simulink model "newrules"  (R2016a)
settings: Solver=VariableStepAuto  StartTime=0.0  StopTime=10.0  RelTol=1e-3
libraries: fuzblock x5, simulink x1
settings Model: Creator=SPDKH  LastModifiedBy=SPDKH

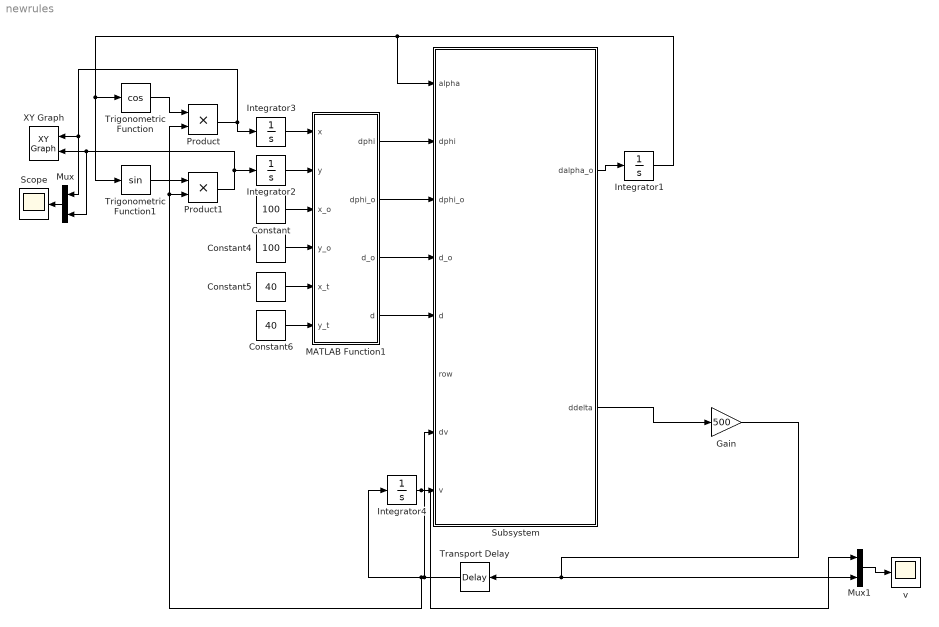
== system newrules ==
  Constant : Constant  Value=100
  Constant4 : Constant  Value=100
  Constant5 : Constant  Value=40
  Constant6 : Constant  Value=40
  Gain : Gain  Gain=500
  Integrator1 : Integrator
  Integrator2 : Integrator
  Integrator3 : Integrator  InitialCondition=30
  Integrator4 : Integrator
  MATLAB Function1 : MATLAB Function  TreatAsAtomicUnit=on
  Mux : Mux  Inputs=2
  Mux1 : Mux  Inputs=2
  Product : Product
  Product1 : Product
  Scope : Scope
  Subsystem : Subsystem
  Transport Delay : TransportDelay
  Trigonometric Function : Trigonometry  Operator=cos
  Trigonometric Function1 : Trigonometry
  XY Graph : simulink/Sinks/XY Graph  xmin=-10  xmax=100  ymin=-10  ymax=100  st=-1
  v : Scope
  wires:
  Subsystem/2(ddelta) -> Gain/1
  Constant/1 -> MATLAB Function1/3(x_o)
  Constant4/1 -> MATLAB Function1/4(y_o)
  Constant5/1 -> MATLAB Function1/5(x_t)
  Constant6/1 -> MATLAB Function1/6(y_t)
  MATLAB Function1/1(dphi) -> Subsystem/2("dphi ")
  MATLAB Function1/2(dphi_o) -> Subsystem/3("dphi_o ")
  MATLAB Function1/3(d_o) -> Subsystem/4(d_o)
  MATLAB Function1/4(d) -> Subsystem/5(d)
  Subsystem/1("dalpha_o ") -> Integrator1/1
  Integrator2/1 -> MATLAB Function1/2(y)
  Integrator3/1 -> MATLAB Function1/1(x)
  Trigonometric Function/1 -> Product/1
  Trigonometric Function1/1 -> Product1/1
  Integrator1/1 -> Subsystem/1(alpha), Trigonometric Function1/1, Trigonometric Function/1
  Product/1 -> Mux/1, XY Graph/1, Integrator3/1
  Product1/1 -> Mux/2, XY Graph/2, Integrator2/1
  Gain/1 -> Mux1/2, Transport Delay/1
  Transport Delay/1 -> Integrator4/1, Product1/2, Product/2, Subsystem/7(dv)
  Mux1/1 -> v/1
  Integrator4/1 -> Mux1/1, Subsystem/8(v)
  Mux/1 -> Scope/1

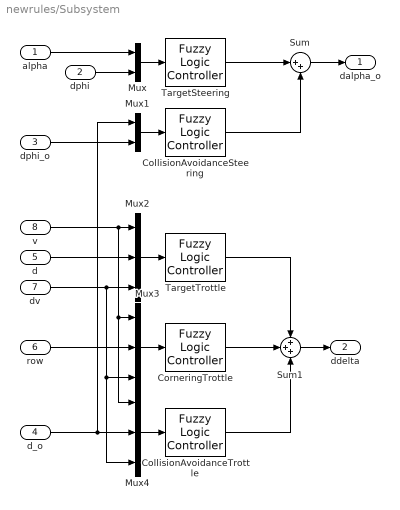
== system newrules/Subsystem ==
  alpha : Inport
  "dphi " : Inport  Port=2
  "dphi_o " : Inport  Port=3
  d_o : Inport  Port=4
  d : Inport  Port=5
  row : Inport  Port=6
  dv : Inport  Port=7
  v : Inport  Port=8
  "CollisionAvoidanceSteering " : fuzblock/Fuzzy Logic  Controller  fis=['CollisionAvoidanceSteering.fis']
  "CollisionAvoidanceTrottle " : fuzblock/Fuzzy Logic  Controller  fis=['CollisionAvoidanceThrottle.fis']
  "CorneringTrottle " : fuzblock/Fuzzy Logic  Controller  fis=['CorneringTrottle.fis']
  Mux : Mux  Inputs=2
  Mux1 : Mux  Inputs=2
  Mux2 : Mux  Inputs=3
  Mux3 : Mux  Inputs=3
  Mux4 : Mux  Inputs=3
  Sum : Sum  Inputs=|++
  Sum1 : Sum  Inputs=+++
  TargetSteering : fuzblock/Fuzzy Logic  Controller  fis=['TargetSteering2.fis']
  TargetTrottle : fuzblock/Fuzzy Logic  Controller  fis=['TargetTrottle.fis']
  "dalpha_o " : Outport
  ddelta : Outport  Port=2
  wires:
  TargetTrottle/1 -> Sum1/1
  "CorneringTrottle "/1 -> Sum1/2
  "CollisionAvoidanceTrottle "/1 -> Sum1/3
  TargetSteering/1 -> Sum/1
  "CollisionAvoidanceSteering "/1 -> Sum/2
  Mux/1 -> TargetSteering/1
  Mux1/1 -> "CollisionAvoidanceSteering "/1
  Mux2/1 -> TargetTrottle/1
  Mux3/1 -> "CorneringTrottle "/1
  Mux4/1 -> "CollisionAvoidanceTrottle "/1
  v/1 -> Mux4/1, Mux3/1, Mux2/1
  d/1 -> Mux2/2
  dv/1 -> Mux4/3, Mux3/3, Mux2/3
  row/1 -> Mux3/2
  d_o/1 -> Mux1/1, Mux4/2
  alpha/1 -> Mux/1
  "dphi "/1 -> Mux/2
  "dphi_o "/1 -> Mux1/2
  Sum/1 -> "dalpha_o "/1
  Sum1/1 -> ddelta/1

== matlab function newrules/MATLAB Function1 ==
  data: dphi output; dphi_o output; d_o output; x input; d output; y input; x_o input; y_o input; x_t input; y_t input
function [dphi,dphi_o,d_o,d] = fcn(x,y,x_o,y_o,x_t,y_t)

 if ((x_t-x) < 0)
     dphi = atan ((y_t-y)/(x_t-x))+pi;
 else 
    dphi = atan ((y_t-y)/(x_t-x));
 end
 
 if ((x_o-x) < 0)
     dphi_o = atan ((y_o-y)/(x_o-x));+pi;
 else 
    dphi_o = atan ((y_o-y)/(x_o-x));
 end


d_o = norm([(x_o-x),(y_o-y)]);
d = norm([(x_t-x),(y_t-y)]);
